simulink model "plant_ss_gainscheduled"  (R2019a)
settings: Solver=VariableStepAuto  StartTime=0.0  StopTime=2000  MaxStep=1  RelTol=1e-3
values from neighbouring files (symbols this model uses):
  M = 20    [initialise_parameters.m]
  rhoA = 20    [initialise_parameters.m]
  UA2 = 6.84    [initialise_parameters.m]
undefined symbols (not defined in the file or in its folder): K_schedule, u0_schedule, X2_schedule
libraries: simulink x2
settings Model: Creator=amah2  LastModifiedBy=kovim
settings DataIOCC: MaxDataPoints=10  SaveOperatingPoint=on  SaveFormat=Array  SignalLogging=off  DSMLogging=off

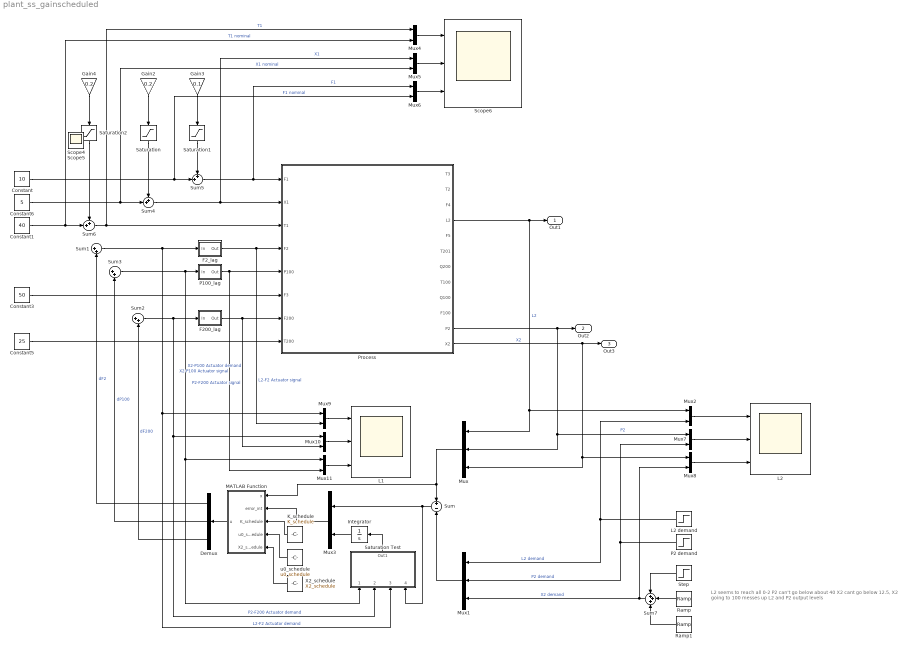
== system plant_ss_gainscheduled ==
  note: L2 seems to reach all 0-2
      | P2 can't go below about 40
      | X2 cant go below 12.5, X2 going to 100 messes up L2 and P2 output levels
  Constant : Constant  Value=10
  Constant1 : Constant  Value=40
  Constant3 : Constant  Value=50
  Constant5 : Constant  Value=25
  Constant6 : Constant  Value=5
  Demux : Demux  Outputs=3
  F200_lag : Subsystem
  F2_lag : Subsystem
  Gain2 : Gain  Gain=0.2
  Gain3 : Gain  Gain=0.1
  Gain4 : Gain  Gain=0.2
  Integrator : Integrator  UpperSaturationLimit=208  LowerSaturationLimit=-208  ZeroCross=off
  "K_schedule " : Constant  Value=K_schedule
  L1 : Scope  NumInputPorts=3
  L2 : Scope  NumInputPorts=3
  L2 demand : Step  Time=10  Before=1  SampleTime=0
  MATLAB Function : MATLAB Function  TreatAsAtomicUnit=on
  Mux : Mux  Inputs=3
  Mux1 : Mux  Inputs=3
  Mux{2..11} (10 alike) : Mux  Inputs=2
  P100_lag : Subsystem
  "P2 demand " : Step  Time=10  Before=50.5  After=50.5  SampleTime=0
  Process : Subsystem
  Ramp : simulink/Sources/Ramp  slope=0  start=100  InitialOutput=0
  Ramp1 : simulink/Sources/Ramp  slope=0  start=110  InitialOutput=0
  Saturation : Saturate  UpperLimit=25  LowerLimit=-5
  Saturation Test : Subsystem
  Saturation1 : Saturate  UpperLimit=2  LowerLimit=-2
  Saturation2 : Saturate  UpperLimit=4  LowerLimit=-4
  Scope6 : Scope  NumInputPorts=3
  Step : Step  Time=50  Before=25  After=25  SampleTime=0
  Sum : Sum  Inputs=+|-
  Sum1 : Sum  Inputs=|++
  Sum2 : Sum  Inputs=|++
  Sum3 : Sum  Inputs=|++
  Sum4 : Sum  Inputs=++|
  Sum5 : Sum  Inputs=++|
  Sum6 : Sum  Inputs=++|
  Sum7 : Sum  Inputs=+++
  X2_schedule : Constant  Value=X2_schedule
  u0_schedule : Constant  Value=u0_schedule
  Out1 : Outport
  Out2 : Outport  Port=2
  Out3 : Outport  Port=3
  Scope4 : Scope
  Scope5 : Scope
  wires:
  Process/4(L2) -> Mux/1, Mux2/1, Out1/1  "L2"
  Constant3/1 -> Process/6(F3)
  Constant5/1 -> Process/8(T200)
  ? -> Sum1/1
  L2 demand/1 -> Mux1/1, Mux2/2  "L2 demand"
  Demux/1 -> Sum1/2  "dF2"
  "P2 demand "/1 -> Mux7/2, Mux1/2  "P2 demand"
  Process/11(P2) -> Out2/1, Mux/2, Mux7/1  "P2"
  Demux/3 -> Sum2/2  "dF200"
  ? -> Sum2/1
  Sum2/1 -> Saturation Test/2(P2-F200 Actuator demand), Mux10/1, F200_lag/1("In ")  "P2-F200 Actuator demand"
  ? -> Sum3/1
  Process/12(X2) -> Out3/1, Mux/3, Mux8/1  "X2"
  Demux/2 -> Sum3/2  "dP100"
  Sum1/1 -> F2_lag/1("In "), Mux9/1, Saturation Test/3(L2-F2 Actuator demand)  "L2-F2 Actuator demand"
  Sum3/1 -> Saturation Test/1(X2-P100 Actuator demand), Mux11/1, P100_lag/1("In ")  "X2-P100 Actuator demand"
  Sum/1 -> Saturation Test/4("Errors to be integrated "), Mux3/1
  Mux/1 -> MATLAB Function/1(x), Sum/1
  Mux1/1 -> Sum/2
  Integrator/1 -> Mux3/2
  F2_lag/1(Out) -> Mux9/2, Process/4(F2)  "L2-F2 Actuator signal"
  P100_lag/1(Out) -> Process/5(P100), Mux11/2  "X2-P100 Actuator signal"
  F200_lag/1(Out) -> Mux10/2, Process/7(F200)  "P2-F200 Actuator signal"
  Gain2/1 -> Saturation/1
  Gain4/1 -> Saturation2/1
  Sum4/1 -> Mux5/1, Process/2(X1)  "X1"
  ? -> Gain2/1
  Sum5/1 -> Mux6/1, Process/1(F1)  "F1"
  Sum6/1 -> Mux4/1, Process/3(T1)  "T1"
  Gain3/1 -> Saturation1/1
  ? -> Gain3/1
  Constant1/1 -> Mux4/2, Sum6/2  "T1 nominal"
  Constant6/1 -> Mux5/2, Sum4/2  "X1 nominal"
  Constant/1 -> Mux6/2, Sum5/2  "F1 nominal"
  ? -> Gain4/1
  Mux6/1 -> Scope6/3
  Mux4/1 -> Scope6/1
  Mux5/1 -> Scope6/2
  Mux3/1 -> MATLAB Function/2(error_int)
  MATLAB Function/1(u) -> Demux/1
  Sum7/1 -> Mux1/3, Mux8/2  "X2 demand"
  Step/1 -> Sum7/1
  Ramp/1 -> Sum7/2
  Ramp1/1 -> Sum7/3
  Mux2/1 -> L2/1
  Mux7/1 -> L2/2
  Mux8/1 -> L2/3
  Mux9/1 -> L1/1
  Mux11/1 -> L1/3
  Mux10/1 -> L1/2
  Saturation1/1 -> Sum5/1
  Saturation/1 -> Sum4/1
  Saturation2/1 -> Sum6/1
  Saturation Test/1(Out1) -> Integrator/1
  "K_schedule "/1 -> MATLAB Function/3(K_schedule)
  X2_schedule/1 -> MATLAB Function/5(X2_schedule)
  u0_schedule/1 -> MATLAB Function/4(u0_schedule)

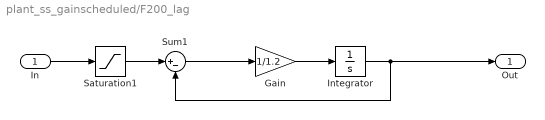
== system plant_ss_gainscheduled/F200_lag ==
  "In " : Inport
  Gain : Gain  Gain=1/1.2
  Integrator : Integrator  InitialCondition=208
  Saturation1 : Saturate  UpperLimit=416  LowerLimit=0  ZeroCross=off
  Sum1 : Sum  Inputs=|+-
  Out : Outport
  wires:
  "In "/1 -> Saturation1/1
  Sum1/1 -> Gain/1
  Gain/1 -> Integrator/1
  Integrator/1 -> Sum1/2, Out/1
  Saturation1/1 -> Sum1/1

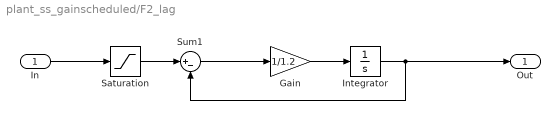
== system plant_ss_gainscheduled/F2_lag ==
  "In " : Inport
  Gain : Gain  Gain=1/1.2
  Integrator : Integrator  InitialCondition=2
  Saturation : Saturate  UpperLimit=4  LowerLimit=0  ZeroCross=off
  Sum1 : Sum  Inputs=|+-
  Out : Outport
  wires:
  "In "/1 -> Saturation/1
  Sum1/1 -> Gain/1
  Gain/1 -> Integrator/1
  Integrator/1 -> Sum1/2, Out/1
  Saturation/1 -> Sum1/1

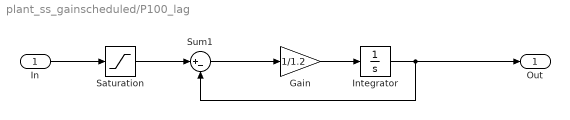
== system plant_ss_gainscheduled/P100_lag ==
  "In " : Inport
  Gain : Gain  Gain=1/1.2
  Integrator : Integrator  InitialCondition=194.7
  Saturation : Saturate  UpperLimit=400  LowerLimit=0  ZeroCross=off
  Sum1 : Sum  Inputs=|+-
  Out : Outport
  wires:
  Sum1/1 -> Gain/1
  Gain/1 -> Integrator/1
  Integrator/1 -> Sum1/2, Out/1
  Saturation/1 -> Sum1/1
  "In "/1 -> Saturation/1

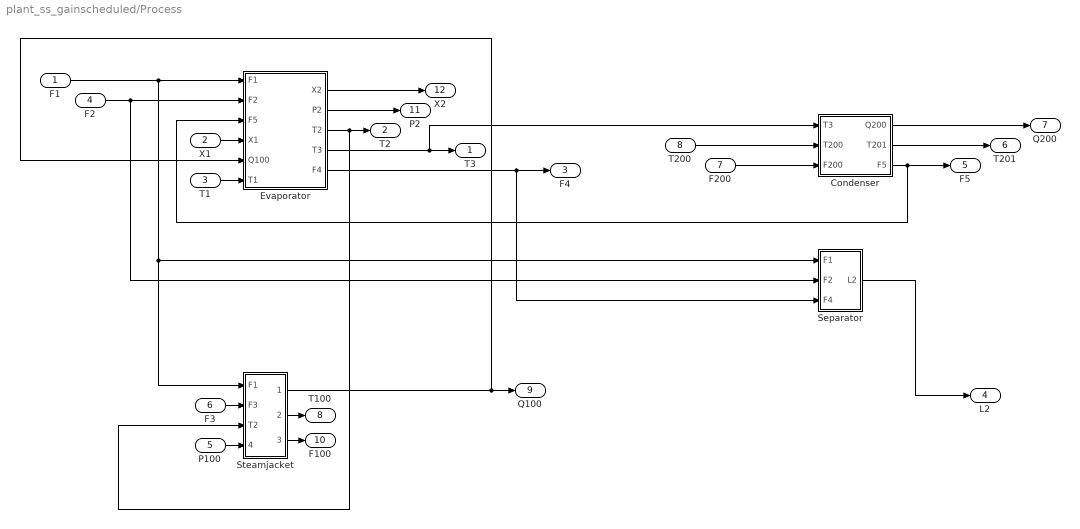
== system plant_ss_gainscheduled/Process ==
  F1 : Inport
  X1 : Inport  Port=2
  T1 : Inport  Port=3
  F2 : Inport  Port=4
  P100 : Inport  Port=5
  F3 : Inport  Port=6
  F200 : Inport  Port=7
  T200 : Inport  Port=8
  Condenser : Subsystem
  Evaporator : Subsystem
  Separator : Subsystem
  Steamjacket : Subsystem
  T3 : Outport  VectorParamsAs1DForOutWhenUnconnected=on
  T2 : Outport  Port=2  VectorParamsAs1DForOutWhenUnconnected=on
  F4 : Outport  Port=3  VectorParamsAs1DForOutWhenUnconnected=on
  L2 : Outport  Port=4  VectorParamsAs1DForOutWhenUnconnected=on
  F5 : Outport  Port=5  VectorParamsAs1DForOutWhenUnconnected=on
  T201 : Outport  Port=6  VectorParamsAs1DForOutWhenUnconnected=on
  Q200 : Outport  Port=7  VectorParamsAs1DForOutWhenUnconnected=on
  T100 : Outport  Port=8  VectorParamsAs1DForOutWhenUnconnected=on
  Q100 : Outport  Port=9  VectorParamsAs1DForOutWhenUnconnected=on
  F100 : Outport  Port=10  VectorParamsAs1DForOutWhenUnconnected=on
  P2 : Outport  Port=11  VectorParamsAs1DForOutWhenUnconnected=on
  X2 : Outport  Port=12  VectorParamsAs1DForOutWhenUnconnected=on
  wires:
  X1/1 -> Evaporator/4(X1)
  T1/1 -> Evaporator/6(T1)
  Evaporator/5("F4 ") -> F4/1, Separator/3("F4 ")
  F1/1 -> Evaporator/1(F1), Steamjacket/1(F1), Separator/1(F1)
  F2/1 -> Evaporator/2(F2), Separator/2(F2)
  F200/1 -> Condenser/3(F200)
  Evaporator/4("T3 ") -> Condenser/1(T3), T3/1
  Evaporator/3("T2 ") -> Steamjacket/3(T2), T2/1
  Evaporator/1(X2) -> X2/1
  Condenser/2(T201) -> T201/1
  Condenser/1(Q200) -> Q200/1
  Steamjacket/1(Q100) -> Evaporator/5(Q100), Q100/1
  Steamjacket/2(T100) -> T100/1
  F3/1 -> Steamjacket/2(F3)
  Steamjacket/3(F100) -> F100/1
  Evaporator/2("P2 ") -> P2/1
  Separator/1(L2) -> L2/1
  Condenser/3(F5) -> F5/1, Evaporator/3(F5)
  P100/1 -> Steamjacket/4(P100)
  T200/1 -> Condenser/2(T200)

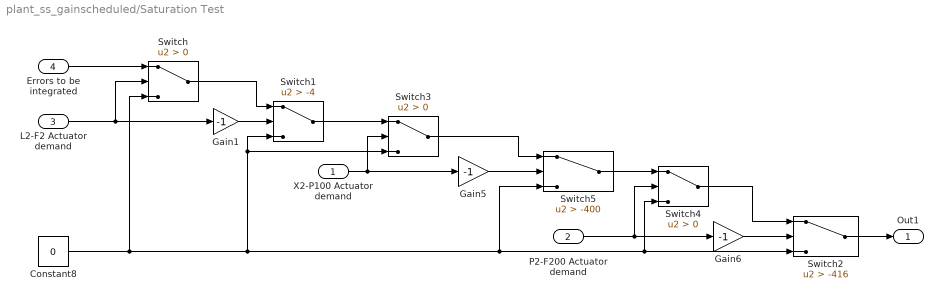
== system plant_ss_gainscheduled/Saturation Test ==
  X2-P100 Actuator demand : Inport
  P2-F200 Actuator demand : Inport  Port=2
  L2-F2 Actuator demand : Inport  Port=3
  "Errors to be integrated " : Inport  Port=4
  Constant8 : Constant  Value=0
  Gain1 : Gain  Gain=-1
  Gain5 : Gain  Gain=-1
  Gain6 : Gain  Gain=-1
  Switch : Switch  Criteria=u2 > Threshold  ZeroCross=off
  Switch1 : Switch  Criteria=u2 > Threshold  Threshold=-4  ZeroCross=off
  Switch2 : Switch  Criteria=u2 > Threshold  Threshold=-416  ZeroCross=off
  Switch3 : Switch  Criteria=u2 > Threshold  ZeroCross=off
  Switch4 : Switch  Criteria=u2 > Threshold  ZeroCross=off
  Switch5 : Switch  Criteria=u2 > Threshold  Threshold=-400  ZeroCross=off
  Out1 : Outport
  wires:
  X2-P100 Actuator demand/1 -> Gain5/1, Switch3/2
  Constant8/1 -> Switch/3, Switch2/3, Switch4/3, Switch5/3, Switch3/3, Switch1/3
  Gain1/1 -> Switch1/2
  Gain6/1 -> Switch2/2
  Switch3/1 -> Switch5/1
  Switch/1 -> Switch1/1
  Gain5/1 -> Switch5/2
  L2-F2 Actuator demand/1 -> Switch/2, Gain1/1
  Switch4/1 -> Switch2/1
  Switch1/1 -> Switch3/1
  Switch5/1 -> Switch4/1
  P2-F200 Actuator demand/1 -> Switch4/2, Gain6/1
  "Errors to be integrated "/1 -> Switch/1
  Switch2/1 -> Out1/1

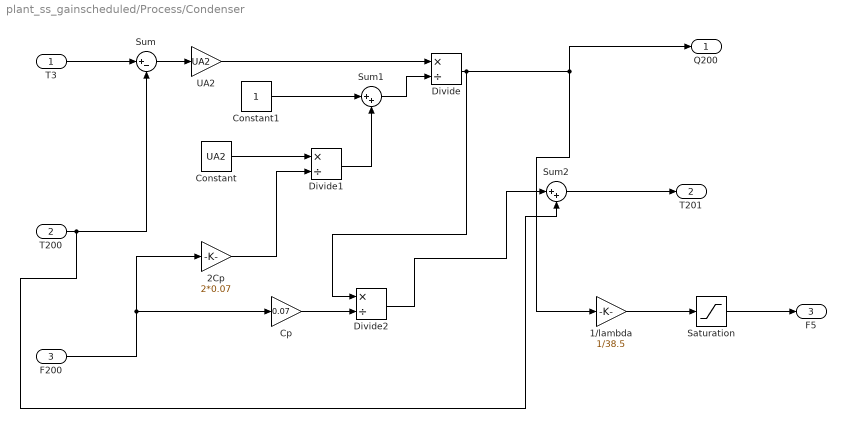
== system plant_ss_gainscheduled/Process/Condenser ==
  T3 : Inport
  T200 : Inport  Port=2
  F200 : Inport  Port=3
  1/lambda : Gain  Gain=1/38.5
  2Cp : Gain  Gain=2*0.07
  Constant : Constant  Value=UA2
  Constant1 : Constant
  Cp : Gain  Gain=0.07
  Divide : Product  Inputs=*/
  Divide1 : Product  Inputs=*/
  Divide2 : Product  Inputs=*/
  Saturation : Saturate  UpperLimit=16  LowerLimit=0
  Sum : Sum  Inputs=|+-
  Sum1 : Sum  Inputs=|++
  Sum2 : Sum  Inputs=|++
  UA2 : Gain  Gain=UA2
  Q200 : Outport  VectorParamsAs1DForOutWhenUnconnected=on
  T201 : Outport  Port=2  VectorParamsAs1DForOutWhenUnconnected=on
  F5 : Outport  Port=3  VectorParamsAs1DForOutWhenUnconnected=on
  wires:
  UA2/1 -> Divide/1
  T200/1 -> Sum/2, Sum2/2
  T3/1 -> Sum/1
  Constant1/1 -> Sum1/1
  Sum2/1 -> T201/1
  Constant/1 -> Divide1/1
  Sum1/1 -> Divide/2
  1/lambda/1 -> Saturation/1
  Divide1/1 -> Sum1/2
  Divide/1 -> Divide2/1, Q200/1, 1/lambda/1
  Sum/1 -> UA2/1
  Divide2/1 -> Sum2/1
  Cp/1 -> Divide2/2
  2Cp/1 -> Divide1/2
  Saturation/1 -> F5/1
  F200/1 -> Cp/1, 2Cp/1

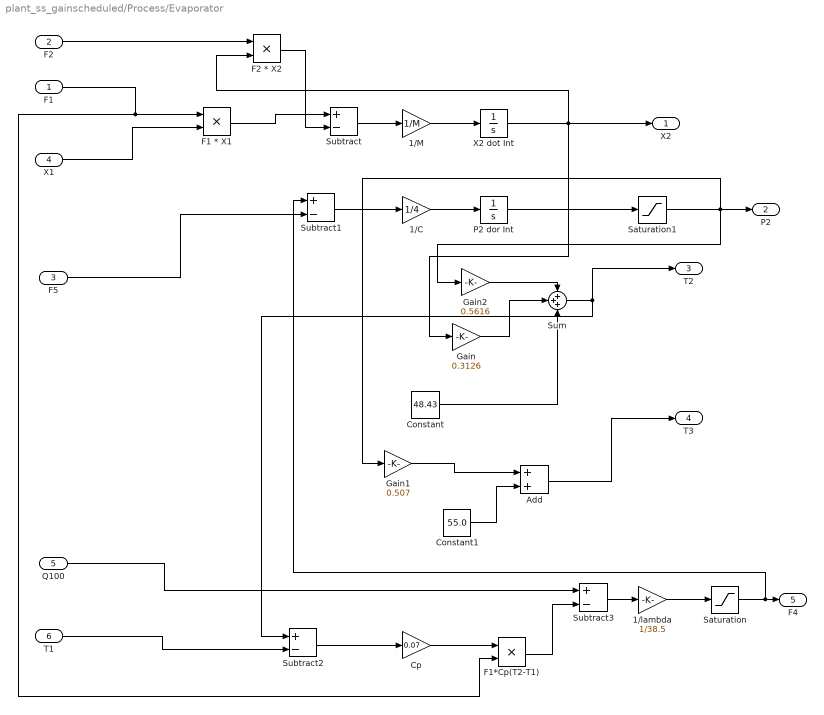
== system plant_ss_gainscheduled/Process/Evaporator ==
  F1 : Inport
  F2 : Inport  Port=2
  F5 : Inport  Port=3
  X1 : Inport  Port=4
  Q100 : Inport  Port=5
  T1 : Inport  Port=6
  1/C : Gain  Gain=1/4
  1/M : Gain  Gain=1/M
  1/lambda : Gain  Gain=1/38.5
  Add : Sum
  Constant : Constant  Value=48.43
  Constant1 : Constant  Value=55.0
  Cp : Gain  Gain=0.07
  F1 * X1 : Product
  F1*Cp(T2-T1) : Product
  F2 * X2 : Product
  Gain : Gain  Gain=0.3126
  Gain1 : Gain  Gain=0.507
  Gain2 : Gain  Gain=0.5616
  P2 dor Int : Integrator  InitialCondition=50.5  ZeroCross=off
  Saturation : Saturate  UpperLimit=16  LowerLimit=0
  Saturation1 : Saturate  UpperLimit=100  LowerLimit=0
  Subtract{,1..3} (4 alike) : Sum  Inputs=+-
  Sum : Sum  Inputs=+++
  X2 dot Int : Integrator  InitialCondition=25  ZeroCross=off
  X2 : Outport
  "P2 " : Outport  Port=2
  "T2 " : Outport  Port=3
  "T3 " : Outport  Port=4
  "F4 " : Outport  Port=5
  wires:
  Constant/1 -> Sum/3
  T1/1 -> Subtract2/2
  X1/1 -> F1 * X1/2
  F1*Cp(T2-T1)/1 -> Subtract3/2
  Sum/1 -> "T2 "/1, Subtract2/1
  P2 dor Int/1 -> Saturation1/1
  Constant1/1 -> Add/2
  Subtract/1 -> 1/M/1
  Subtract2/1 -> Cp/1
  1/lambda/1 -> Saturation/1
  Q100/1 -> Subtract3/1
  Cp/1 -> F1*Cp(T2-T1)/1
  Subtract1/1 -> 1/C/1
  1/C/1 -> P2 dor Int/1
  Gain2/1 -> Sum/1
  1/M/1 -> X2 dot Int/1
  F1 * X1/1 -> Subtract/1
  F2 * X2/1 -> Subtract/2
  X2 dot Int/1 -> X2/1, Gain/1, F2 * X2/2
  F2/1 -> F2 * X2/1
  Gain/1 -> Sum/2
  Add/1 -> "T3 "/1
  Gain1/1 -> Add/1
  F5/1 -> Subtract1/2
  F1/1 -> F1 * X1/1, F1*Cp(T2-T1)/2
  Subtract3/1 -> 1/lambda/1
  Saturation/1 -> "F4 "/1, Subtract1/1
  Saturation1/1 -> "P2 "/1, Gain2/1, Gain1/1

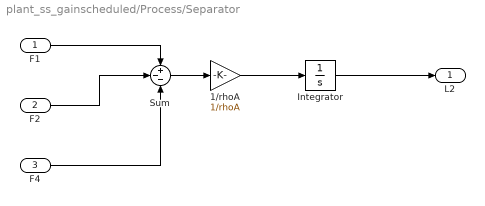
== system plant_ss_gainscheduled/Process/Separator ==
  F1 : Inport
  F2 : Inport  Port=2
  "F4 " : Inport  Port=3
  "1/rhoA " : Gain  Gain=1/rhoA
  Integrator : Integrator  InitialCondition=1  LimitOutput=on  UpperSaturationLimit=2  LowerSaturationLimit=0  ZeroCross=off
  Sum : Sum  Inputs=+--
  L2 : Outport
  wires:
  "F4 "/1 -> Sum/3
  F1/1 -> Sum/1
  F2/1 -> Sum/2
  "1/rhoA "/1 -> Integrator/1
  Sum/1 -> "1/rhoA "/1
  Integrator/1 -> L2/1

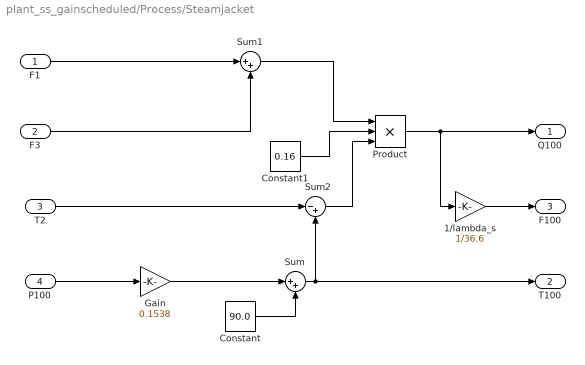
== system plant_ss_gainscheduled/Process/Steamjacket ==
  F1 : Inport
  F3 : Inport  Port=2
  T2 : Inport  Port=3
  P100 : Inport  Port=4
  1/lambda_s : Gain  Gain=1/36.6
  Constant : Constant  Value=90.0
  Constant1 : Constant  Value=0.16
  Gain : Gain  Gain=0.1538
  Product : Product  Inputs=3
  Sum : Sum  Inputs=|++
  Sum1 : Sum  Inputs=|++
  Sum2 : Sum  Inputs=|-+
  Q100 : Outport  VectorParamsAs1DForOutWhenUnconnected=on
  T100 : Outport  Port=2  VectorParamsAs1DForOutWhenUnconnected=on
  F100 : Outport  Port=3  VectorParamsAs1DForOutWhenUnconnected=on
  wires:
  Sum/1 -> T100/1, Sum2/2
  Sum2/1 -> Product/3
  1/lambda_s/1 -> F100/1
  Gain/1 -> Sum/1
  Product/1 -> Q100/1, 1/lambda_s/1
  T2/1 -> Sum2/1
  F3/1 -> Sum1/2
  Sum1/1 -> Product/1
  Constant1/1 -> Product/2
  F1/1 -> Sum1/1
  Constant/1 -> Sum/2
  P100/1 -> Gain/1

== matlab function plant_ss_gainscheduled/MATLAB Function ==
  data: x input; error_int input; u output; K_schedule input; u0_schedule input; X2_schedule input
function u = fcn(x, error_int, K_schedule, u0_schedule, X2_schedule)
    X2 = x(3);
    
    if X2 > max(X2_schedule)
        X2 = max(X2_schedule);
    elseif X2 < min(X2_schedule)
        X2 = min(X2_schedule);
    end
    
    u0 = interp1(X2_schedule, u0_schedule, X2);
    K = interp1(X2_schedule, K_schedule, X2);
    
    u0 = permute(u0, [2 1]);
    K = permute(K, [2 3 1]);
    
    du = K*error_int;
    u = u0 + du;
    
    x
    error_int
    K
    u
